simulink model "System_without_motor"  (R2018a)
settings: Solver=VariableStepAuto  StartTime=0.0  StopTime=10.0  RelTol=1e-3
settings Model: Creator=Zeljko  LastModifiedBy=Zeljko

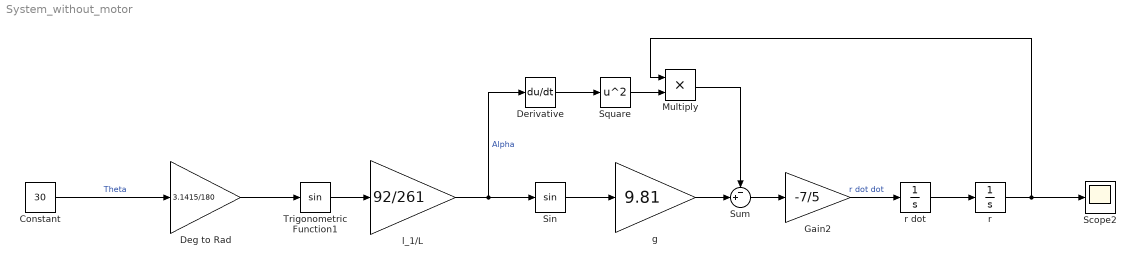
== system System_without_motor ==
  Constant : Constant  Value=30
  Deg to Rad : Gain  Gain=3.1415/180
  Derivative : Derivative
  Gain2 : Gain  Gain=-7/5
  Multiply : Product
  Scope2 : Scope
  Sin : Trigonometry
  Square : Math  Operator=square  SaturateOnIntegerOverflow=on
  Sum : Sum  Inputs=-+|
  Trigonometric Function1 : Trigonometry
  g : Gain  Gain=9.81
  l_1/L : Gain  Gain=92/261
  r : Integrator  InitialCondition=100
  r dot : Integrator
  wires:
  Trigonometric Function1/1 -> l_1/L/1
  Constant/1 -> Deg to Rad/1  "Theta"
  Deg to Rad/1 -> Trigonometric Function1/1
  l_1/L/1 -> Derivative/1, Sin/1  "Alpha"
  Sin/1 -> g/1
  g/1 -> Sum/2
  Sum/1 -> Gain2/1
  r dot/1 -> r/1
  r/1 -> Multiply/1, Scope2/1
  Derivative/1 -> Square/1
  Square/1 -> Multiply/2
  Multiply/1 -> Sum/1
  Gain2/1 -> r dot/1  "r dot dot"
